simulink model "HW6_JamesWilkinson2"  (R2025b)
settings: Solver=VariableStepAuto  StartTime=0.0  StopTime=10  RelTol=1e-3
values from neighbouring files (symbols this model uses):
  Air_mdot = AirFlow(j)    [All_Conditions.m]
  HeatRate = 10^8    (= 100000000)    [All_Conditions.m]    (also in VariedFuelRate.m = HeatRate_vec(i))
libraries: fl_lib x22, nesl_utility x22, SimscapeFluids_lib x2
settings Model: Creator=james  LastModifiedBy=james

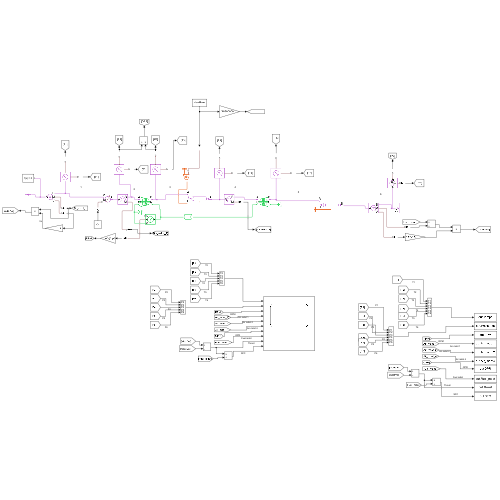
[thumbnail: Simulink's stored preview of the top-level diagram]
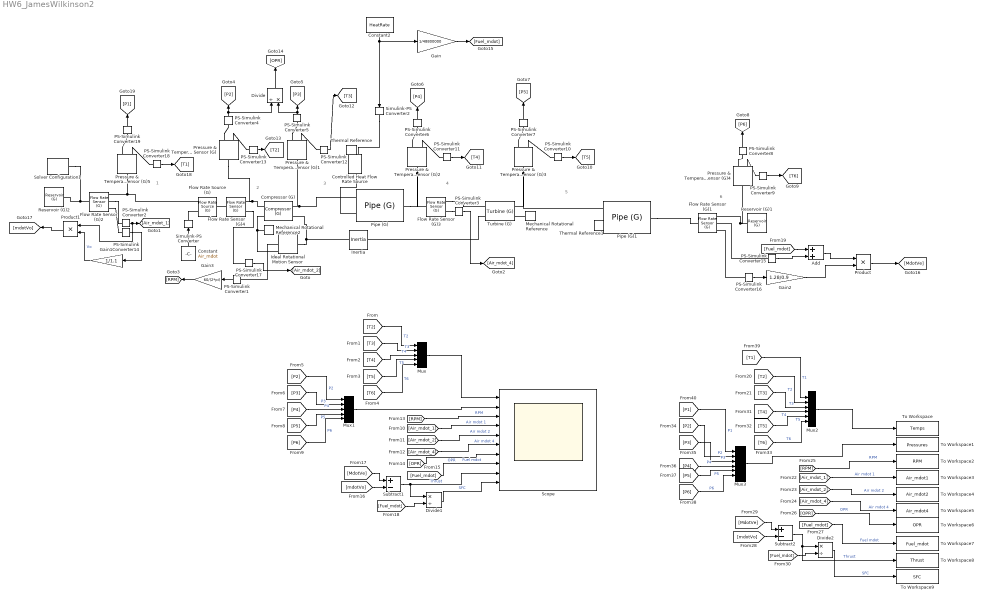
== system HW6_JamesWilkinson2 ==
  note: 6
  note: 5
  note: 4
  note: 3
  note: 2
  note: 1
  Add : Sum
  Compressor (G) : SimscapeFluids_lib/Gas/Turbomachinery/Compressor (G)  parameterization=fluids.gas.turbomachinery.enum.CompressorParameterization.Analytical  NDes=10000 rpm  piDes=DesignedPR  mdotDes=33 kg/s  efficiencyType=fluids.gas.turbomachinery.enum.EfficiencyType.Analytical  efficiencyValue=0.8  etaMax=0.887  etaMin=0.5  mdotMaxEff=30 kg/s  piMaxEff=7  omega_TLU=[5000, 6000, 7000, 7500, 8000, 8500, 9000, 9500, 10000, 11000] rpm  beta_TLU=0 : 1 / 6 : 1  pr_TLU=[1.369, 1.459, 1.587, 1.654, 1.734, 1.775, 1.82; 1.918, 2.075, 2.229, 2.318, 2.405, 2.456, 2.481; 2.706, 2.966, 3.168, 3.334, 3.404, 3.445, 3.435; 3.203, 3.533, 3.833, 4.021, 4.127, 4.135, 4.066; 3.782, 4.222, 4.565, 4.867, 5.065, 5.07, 4.934; 4.302, 4.861, 5.285, 5.821, 6.161, 6.334, 6.142; 4.841, 5.445, 5.988, 6.628, 7.222, 7.623, 7.573; 5.358, 5.997, 6.589, 7.334, 8.012, 8.668, 9; 5.851, 6.491, 7.124, 7.982, 8.754, 9.57, 9.814; 6.707, 7.321, 8.034, 9.047, 9.94, 10.834, 10.998]  mdot_TLU=[10.45, 10.203, 9.784, 9.526, 9.144, 8.947, 8.615; 13.315, 13.018, 12.525, 11.984, 11.455, 11.086, 10.914; 17.601, 17.204, 16.502, 15.8, 14.903, 14.179, 13.184; 20.331, 19.983, 19.39, 18.492, 17.435, 16.293, 14.895; 23.466, 23.092, 22.572, 21.807, 20.687, 19.3, 17.682; 26.295, 26.091, 25.766, 25.28, 24.453, 23.26, 21.311; 29.013, 28.747, 28.641, 28.412, 28.06, 27.098, 25.306; 31.424, 31.379, 31.273, 31.103, 30.849, 30.484, 29.718; 33.688, 33.606, 33.561, 33.513, 33.392, 33.258, 33.059; 37.678, 37.621, 37.575, 37.598, 37.501, 37.415, 37.413] kg/s  eta_TLU=[.68, .69, .695, .7, .701, .705, .704; .7, .725, .75, .755, .745, .73, .725; .77, .795, .81, .805, .78, .765, .745; .795, .812, .825, .82, .805, .78, .75; .82, .837, .848, .849, .835, .805, .78; .83, .845, .856, .86, .855, .84, .8; .83, .848, .859, .869, .86, .852, .83; .828, .845, .857, .869, .862, .855, .85; .806, .83, .85, .86, .859, .857, .853; .79, .8, .82, .835, .845, .848, .849]  SMFault=simscape.enum.assert.action.none  a=1.5  b=5  k=0.03  c=3  d=4  cCap=15  dCap=1  p_reference=0.101325 MPa  T_reference=288.15 K  mechanical_efficiency=0.9  area_A=1.28 m^2  area_B=1 m^2
      settings: InternalSimscapePortConfiguration="{\"Bottom\":[],\"Left\":[{\"id\":\"A\",\"label\":\"A\",\"type\":\"foundation.gas.gas\"},{\"id\":\"C\",\"label\":\"C\",\"type\":\"foundation.mechanical.rotational.rotational\"}],\"Right\":[{\"id\":\"B\",\"label\":\"B\",\"type\":\"foundation.gas.gas\"},{\"id\":\"R\",\"label\":\"R\",\"type\":\"foundation.mechanical.rotational.rotational\"}],\"Top\":[]}"
  Constant : Constant  Value=Air_mdot
  Constant2 : Constant  Value=HeatRate
  Controlled Heat Flow Rate Source : fl_lib/Thermal/Thermal Sources/Controlled Heat Flow Rate Source
  Divide : Product  Inputs=/*
  Divide1 : Product  Inputs=*/
  Divide2 : Product  Inputs=*/
  Flow Rate Sensor (G)1 : fl_lib/Gas/Sensors/Flow Rate Sensor (G)  mass_flow_measure=true  volumetric_flow_measure=true  volumetric_flow_conditions=foundation.enum.volumetric_flow_conditions.actual  p_std=0.101325 MPa  T_std=20 degC  energy_flow_measure=false
      settings: InternalSimscapePortConfiguration="{\"Bottom\":[],\"Left\":[{\"id\":\"A\",\"label\":\"A\",\"type\":\"foundation.gas.gas\"}],\"Right\":[{\"id\":\"B\",\"label\":\"B\",\"type\":\"foundation.gas.gas\"},{\"id\":\"M\",\"label\":\"M\",\"type\":\"output\"},{\"id\":\"V\",\"label\":\"V\",\"type\":\"output\"}],\"Top\":[]}"
  Flow Rate Sensor (G)2 : fl_lib/Gas/Sensors/Flow Rate Sensor (G)  mass_flow_measure=true  volumetric_flow_measure=true  volumetric_flow_conditions=foundation.enum.volumetric_flow_conditions.actual  p_std=0.101325 MPa  T_std=20 degC  energy_flow_measure=false
      settings: InternalSimscapePortConfiguration="{\"Bottom\":[],\"Left\":[{\"id\":\"A\",\"label\":\"A\",\"type\":\"foundation.gas.gas\"}],\"Right\":[{\"id\":\"B\",\"label\":\"B\",\"type\":\"foundation.gas.gas\"},{\"id\":\"M\",\"label\":\"M\",\"type\":\"output\"},{\"id\":\"V\",\"label\":\"V\",\"type\":\"output\"}],\"Top\":[]}"
  Flow Rate Sensor (G)3 : fl_lib/Gas/Sensors/Flow Rate Sensor (G)  mass_flow_measure=true  volumetric_flow_measure=false  volumetric_flow_conditions=foundation.enum.volumetric_flow_conditions.actual  p_std=0.101325 MPa  T_std=20 degC  energy_flow_measure=false
      settings: InternalSimscapePortConfiguration="{\"Bottom\":[],\"Left\":[{\"id\":\"A\",\"label\":\"A\",\"type\":\"foundation.gas.gas\"}],\"Right\":[{\"id\":\"B\",\"label\":\"B\",\"type\":\"foundation.gas.gas\"},{\"id\":\"M\",\"label\":\"M\",\"type\":\"output\"}],\"Top\":[]}"
  Flow Rate Sensor (G)4 : fl_lib/Gas/Sensors/Flow Rate Sensor (G)  mass_flow_measure=true  volumetric_flow_measure=false  volumetric_flow_conditions=foundation.enum.volumetric_flow_conditions.actual  p_std=0.101325 MPa  T_std=20 degC  energy_flow_measure=false
      settings: InternalSimscapePortConfiguration="{\"Bottom\":[],\"Left\":[{\"id\":\"A\",\"label\":\"A\",\"type\":\"foundation.gas.gas\"}],\"Right\":[{\"id\":\"B\",\"label\":\"B\",\"type\":\"foundation.gas.gas\"},{\"id\":\"M\",\"label\":\"M\",\"type\":\"output\"}],\"Top\":[]}"
  Flow Rate Source (G) : fl_lib/Gas/Sources/Flow Rate Source (G)  source_type=foundation.enum.constant_controlled.controlled  flow_type=foundation.enum.mass_volumetric_flow.mass  mass_flow=0 kg/s  volumetric_flow=0 m^3/s  volumetric_flow_conditions=foundation.enum.volumetric_flow_conditions.actual  p_std=0.101325 MPa  T_std=20 degC  power_spec=foundation.enum.power_spec.isentropic  area_A=1.1 m^2  area_B=1.28 m^2
      settings: InternalSimscapePortConfiguration="{\"Bottom\":[],\"Left\":[{\"id\":\"A\",\"label\":\"A\",\"type\":\"foundation.gas.gas\"},{\"id\":\"M\",\"label\":\"M\",\"type\":\"input\"}],\"Right\":[{\"id\":\"B\",\"label\":\"B\",\"type\":\"foundation.gas.gas\"}],\"Top\":[]}"
  Gain : Gain  Gain=1/48800000
  Gain1 : Gain  Gain=1/1.1
  Gain2 : Gain  Gain=1.28/0.9
  Gain3 : Gain  Gain=60/(2*pi)
  Ideal Rotational Motion Sensor : fl_lib/Mechanical/Mechanical Sensors/Ideal Rotational Motion Sensor  reference=foundation.enum.MeasurementReference.difference  acceleration_port=false  velocity_port=true  position_port=true  wrap_angle=false  offset=0 rad
  Inertia : fl_lib/Mechanical/Rotational Elements/Inertia  inertia=0.01 kg*m^2  num_ports=foundation.enum.numPorts2.two  w_specify=on  w_priority=High  w=1400 rad/s  w_nominal_specify=off  w_nominal_value=1  w_nominal_unit=rad/s  t_specify=off  t_priority=None  t=0 N*m  t_nominal_specify=off  t_nominal_value=1  t_nominal_unit=N*m
      settings: InternalSimscapePortConfiguration="{\"Bottom\":[],\"Left\":[{\"id\":\"I\",\"label\":\"\",\"type\":\"foundation.mechanical.rotational.rotational\"}],\"Right\":[{\"id\":\"J\",\"label\":\"\",\"type\":\"foundation.mechanical.rotational.rotational\"}],\"Top\":[]}"
  Mechanical Rotational Reference : fl_lib/Mechanical/Rotational Elements/Mechanical Rotational Reference
  Mechanical Rotational Reference2 : fl_lib/Mechanical/Rotational Elements/Mechanical Rotational Reference
  Mux : Mux  Inputs=5
      settings: DisplayOption=signals
  Mux1 : Mux  Inputs=5
      settings: DisplayOption=signals
  Mux2 : Mux  Inputs=6
      settings: DisplayOption=signals
  Mux3 : Mux  Inputs=6
      settings: DisplayOption=signals
  PS-Simulink Converter{1..19} (19 alike) : nesl_utility/PS-Simulink Converter  PhysicalDomain=network_engine_domain  SubClassName=ps_output  LeftPortType=input  RightPortType=output  PseudoPeriodic=off  Frequencies=[]  VectorFormat=inherit  Unit=inherit  AffineConversion=off
  Pipe (G) : fl_lib/Gas/Elements/Pipe (G)  length=0.5 m  area=1 m^2  Dh=4/(pi) m  length_add=0.1 m  roughness=15e-6 m  Re_lam=2000  Re_tur=4000  shape_factor=64  Nu_lam=3.66  dynamic_compressibility=true  inertia=false  p_init=.5 MPa  p_init_priority=foundation.enum.Priority.High  T_init=500 K  T_init_priority=foundation.enum.Priority.High  mdot_init=0 kg/s  mdot_init_priority=foundation.enum.Priority.High  p_nominal=0.101325 MPa  T_nominal=293.15 K
  Pipe (G)1 : fl_lib/Gas/Elements/Pipe (G)  length=0.5 m  area=1.28 m^2  Dh=sqrt(1.28/pi*4) m  length_add=0.1 m  roughness=15e-6 m  Re_lam=2000  Re_tur=4000  shape_factor=64  Nu_lam=3.66  dynamic_compressibility=true  inertia=false  p_init=0.101325 MPa  p_init_priority=foundation.enum.Priority.High  T_init=293.15 K  T_init_priority=foundation.enum.Priority.High  mdot_init=0 kg/s  mdot_init_priority=foundation.enum.Priority.High  p_nominal=0.101325 MPa  T_nominal=293.15 K
  Pressure & Temperature Sensor (G){,1..5} (6 alike) : fl_lib/Gas/Sensors/Pressure & Temperature Sensor (G)  reference=foundation.enum.MeasurementReference.absolute  pressure=true  pressure_spec=foundation.enum.PressureMeasementSpec.Absolute  temperature=true
      settings: InternalSimscapePortConfiguration="{\"Bottom\":[{\"id\":\"T\",\"label\":\"T\",\"type\":\"output\"}],\"Left\":[{\"id\":\"A\",\"label\":\"A\",\"type\":\"foundation.gas.gas\"}],\"Right\":[{\"id\":\"Pa\",\"label\":\"Pa\",\"type\":\"output\"}],\"Top\":[]}"
  Product : Product
  Product1 : Product
  Reservoir (G)1 : fl_lib/Gas/Elements/Reservoir (G)  pressure_spec=foundation.enum.pressure_spec.specified  reservoir_pressure=Pressure MPa  reservoir_temperature=Temp K  area_A=1.28 m^2
  Reservoir (G)2 : fl_lib/Gas/Elements/Reservoir (G)  pressure_spec=foundation.enum.pressure_spec.specified  reservoir_pressure=Pressure MPa  reservoir_temperature=Temp K  area_A=1.1 m^2
  Scope : Scope  NumInputPorts=10
      settings: ActiveDisplayYMinimum=-67303.986075745488  ActiveDisplayYMaximum=721507.2488354966
  Simulink-PS Converter : nesl_utility/Simulink-PS Converter  PhysicalDomain=network_engine_domain  SubClassName=ps_input  LeftPortType=input  RightPortType=output  PseudoPeriodic=off  Frequencies=[]  NoiseDistribution=none  NoiseParameters=[]  Unit=1  AffineConversion=off  FilteringAndDerivatives=provide  SimscapeFilterOrder=1  InputFilterTimeConstant=0.001  UdotUserProvided=0
  Simulink-PS Converter2 : nesl_utility/Simulink-PS Converter  PhysicalDomain=network_engine_domain  SubClassName=ps_input  LeftPortType=input  RightPortType=output  PseudoPeriodic=off  Frequencies=[]  NoiseDistribution=none  NoiseParameters=[]  Unit=1  AffineConversion=off  FilteringAndDerivatives=provide  SimscapeFilterOrder=1  InputFilterTimeConstant=0.001  UdotUserProvided=0
  Solver Configuration1 : nesl_utility/Solver Configuration  PhysicalDomain=network_engine_domain  SubClassName=solver  LeftPortType=input  RightPortType=generic  Tones=[]  Harmonics=[]  SimulateNoise=off  Profile=off  UseLocalSampling=off  EnableSwitchedLinearOptims=on  FrequencyDomain=off  UseCCode=off  RelTol=0.001  AbsTol=0.001  MinStep=1e-09  ToWorkspace=off  RevertToSquareIcSolve=off  NumHomotopyIterations=100  PhasorMode=off  PhasorModeNumHarmonics=1  ConsistencySolver=NEWTON_XTOL_AFTER_FTOL  IndexReductionMethod=DerivativeReplacement  DoDC=off  ResidualTolerance=1e-09  ConsistencyTolSource=GLOBAL  ConsistencyAbsTol=0.001  ConsistencyRelTol=0.001  ConsistencyTolFactor=0.001  UseLocalSolver=off  LocalSolverChoice=NE_BACKWARD_EULER_ADVANCER  ResolveIndetEquations=on  FunctionEvalNumThread=1  LocalSolverSampleTime=0.001  DoFixedCost=off  MaxNonlinIter=3  MaxModeIter=2  ComputeImpulses=off  ImpulseIterations=2  LinearAlgebra=auto  LinearAlgebraNumThread=0  EquationFormulation=NE_TIME_EF  DelaysMemoryBudget=1024  AutomaticFiltering=on  FilteringTimeConstant=0.001  PartitionStorageMethod=AS_NEEDED  PartitionMemoryBudget=1024  PartitionMethod=ROBUST  MultibodyUseLocalSolver=off  MultibodyLocalSolverChoice=ODE1  MultibodyLocalSolverSampleTime=0.001
  Subtract1 : Sum  Inputs=+-
  Subtract2 : Sum  Inputs=+-
  Thermal Reference : fl_lib/Thermal/Thermal Elements/Thermal Reference
  Thermal Reference1 : fl_lib/Thermal/Thermal Elements/Thermal Reference
  To Workspace : ToWorkspace  VariableName=Temps  SaveFormat=Timeseries  SampleTime=-1
  To Workspace1 : ToWorkspace  VariableName=Pressures  SaveFormat=Timeseries  SampleTime=-1
  To Workspace2 : ToWorkspace  VariableName=RPM  SaveFormat=Timeseries  SampleTime=-1
  To Workspace3 : ToWorkspace  VariableName=Air_mdot1  SaveFormat=Timeseries  SampleTime=-1
  To Workspace4 : ToWorkspace  VariableName=Air_mdot2  SaveFormat=Timeseries  SampleTime=-1
  To Workspace5 : ToWorkspace  VariableName=Air_mdot4  SaveFormat=Timeseries  SampleTime=-1
  To Workspace6 : ToWorkspace  VariableName=OPR  SaveFormat=Timeseries  SampleTime=-1
  To Workspace7 : ToWorkspace  VariableName=Fuel_mdot  SaveFormat=Timeseries  SampleTime=-1
  To Workspace8 : ToWorkspace  VariableName=Thrust  SaveFormat=Timeseries  SampleTime=-1
  To Workspace9 : ToWorkspace  VariableName=SFC  SaveFormat=Timeseries  SampleTime=-1
  Turbine (G) : SimscapeFluids_lib/Gas/Turbomachinery/Turbine (G)  parameterization=fluids.gas.turbomachinery.enum.TurbineParameterization.Analytical  omega_TLU_2=[5000, 6000, 7000, 8000, 9000, 10000, 11000] rpm  variable_nozzle=false  min_nozzle_opening=1e-3  max_nozzle_opening=1  pr_nom=2  mdot_nom=48 kg/s  pr_mdot_TLU=[1.251, 1.345, 1.442, 1.521, 1.596, 1.692, 1.849, 1.972, 2.1, 2.173, 2.259, 2.3424]  mdot_TLU=[39.439, 43.01, 45.556, 46.801, 47.792, 48.388, 48.634, 48.67, 48.689, 48.747, 48.825, 48.912] kg/s  pr_mdot_TLU_2=[1.217, 1.285, 1.323, 1.363, 1.402, 1.427, 1.495, 1.545, 1.6, 1.687, 1.747, 1.8074; 1.231, 1.302, 1.356, 1.404, 1.443, 1.473, 1.525, 1.577, 1.635, 1.709, 1.782, 1.845; 1.242, 1.328, 1.388, 1.437, 1.528, 1.617, 1.704, 1.811, 1.915, 1.979, 2.053, 2.1226; 1.244, 1.339, 1.417, 1.465, 1.528, 1.584, 1.692, 1.787, 1.899, 2, 2.075, 2.1492; 1.245, 1.34, 1.425, 1.492, 1.546, 1.684, 1.748, 1.882, 1.987, 2.084, 2.167, 2.2458; 1.251, 1.345, 1.442, 1.521, 1.596, 1.692, 1.849, 1.972, 2.1, 2.173, 2.259, 2.3424; 1.248, 1.348, 1.447, 1.516, 1.581, 1.651, 1.749, 1.839, 1.93, 2.024, 2.154, 2.242]  mdot_TLU_2=[40.403, 44.417, 46.653, 47.966, 48.97, 49.544, 50.001, 50.081, 50.086, 50.095, 50.09, 50.0922; 40.044, 43.754, 46.125, 47.626, 48.513, 49.105, 49.481, 49.58, 49.597, 49.624, 49.638, 49.633; 39.941, 43.795, 46.017, 47.335, 48.795, 49.199, 49.279, 49.27, 49.248, 49.23, 49.255, 49.2428; 39.896, 43.512, 45.914, 47.061, 48.011, 48.558, 48.943, 49.042, 49.069, 49.01, 49.046, 49.0266; 39.524, 42.934, 45.686, 46.743, 47.715, 48.67, 48.777, 48.836, 48.876, 48.836, 48.845, 48.8184; 39.439, 43.01, 45.556, 46.801, 47.792, 48.388, 48.634, 48.67, 48.639, 48.647, 48.625, 48.5912; 39.502, 42.849, 45.336, 46.385, 47.312, 47.877, 48.222, 48.397, 48.459, 48.482, 48.455, 48.414] kg/s  efficiency_constant=0.8  pr_eta_TLU=[1.252, 1.328, 1.425, 1.544, 1.642, 1.757, 1.873, 2.005, 2.1, 2.204, 2.248, 2.28]  eta_TLU=[.559, .61, .673, .741, .788, .835, .869, .895, .908, .899, .854, .751]  pr_eta_TLU_2=[1.224, 1.246, 1.292, 1.387, 1.457, 1.534, 1.61, 1.686, 1.743, 1.79, 1.871, 1.914; 1.237, 1.25, 1.28, 1.369, 1.459, 1.553, 1.629, 1.716, 1.799, 1.846, 1.927, 1.97; 1.241, 1.255, 1.283, 1.326, 1.401, 1.509, 1.591, 1.704, 1.806, 1.913, 1.994, 2.037; 1.25, 1.265, 1.308, 1.364, 1.456, 1.532, 1.637, 1.739, 1.851, 1.934, 2.042, 2.085; 1.281, 1.314, 1.371, 1.425, 1.498, 1.574, 1.647, 1.749, 1.878, 1.979, 2.091, 2.18; 1.252, 1.328, 1.425, 1.544, 1.642, 1.757, 1.873, 2.005, 2.1, 2.204, 2.248, 2.28; 1.382, 1.43, 1.495, 1.586, 1.688, 1.791, 1.887, 1.99, 2.079, 2.158, 2.249, 2.36]  eta_TLU_2=[.72, .754, .759, .739, .714, .679, .643, .603, .554, .524, .494, .48; .716, .757, .794, .819, .812, .788, .761, .728, .692, .662, .632, .618; .629, .691, .775, .831, .858, .869, .859, .842, .816, .782, .752, .738; .594, .668, .757, .804, .857, .883, .892, .893, .884, .865, .835, .821; .664, .72, .779, .823, .858, .883, .897, .905, .904, .896, .883, .868; .559, .61, .673, .741, .788, .835, .869, .895, .908, .899, .854, .751; .718, .785, .824, .855, .882, .9, .908, .906, .884, .857, .804, .701]  p_reference=0.101325 MPa  T_reference=288.15 K  mechanical_efficiency=0.9  area_A=1 m^2  area_B=1.28 m^2
      settings: InternalSimscapePortConfiguration="{\"Bottom\":[],\"Left\":[{\"id\":\"A\",\"label\":\"A\",\"type\":\"foundation.gas.gas\"},{\"id\":\"R\",\"label\":\"R\",\"type\":\"foundation.mechanical.rotational.rotational\"}],\"Right\":[{\"id\":\"B\",\"label\":\"B\",\"type\":\"foundation.gas.gas\"},{\"id\":\"C\",\"label\":\"C\",\"type\":\"foundation.mechanical.rotational.rotational\"}],\"Top\":[]}"
  wires:
  Constant/1 -> Simulink-PS Converter/1
  PS-Simulink Converter8/1 -> [P6]
  PS-Simulink Converter9/1 -> [T6]
  Add/1 -> Product/1
  Gain2/1 -> Product/2
  PS-Simulink Converter15/1 -> Add/2
  Product/1 -> [MdotVe]
  [Fuel_mdot] -> Add/1
  PS-Simulink Converter16/1 -> Gain2/1
  PS-Simulink Converter10/1 -> [T5]
  PS-Simulink Converter7/1 -> [P5]
  PS-Simulink Converter6/1 -> [P4]
  PS-Simulink Converter11/1 -> [T4]
  PS-Simulink Converter12/1 -> [T3]
  Divide/1 -> [OPR]
  PS-Simulink Converter4/1 -> Divide/1, [P2]
  PS-Simulink Converter5/1 -> Divide/2, [P3]
  PS-Simulink Converter13/1 -> [T2]
  PS-Simulink Converter14/1 -> Gain1/1
  PS-Simulink Converter2/1 -> Product1/1, [Air_mdot_1]
  Gain1/1 -> Product1/2  "Vo"
  Product1/1 -> [mdotVo]
  PS-Simulink Converter1/1 -> Gain3/1
  Gain3/1 -> [RPM]
  PS-Simulink Converter3/1 -> [Air_mdot_4]
  PS-Simulink Converter17/1 -> [Air_mdot_2]
  Subtract1/1 -> Divide1/1, Scope/9  "Thrust"
  [Fuel_mdot] -> Scope/8  "Fuel mdot"
  [Air_mdot_4] -> Scope/6  "Air mdot 4"
  [T3] -> Mux/2  "T3"
  [OPR] -> Scope/7  "OPR"
  [P5] -> Mux1/4  "P5"
  [P2] -> Mux1/1  "P2"
  [T6] -> Mux/5  "T6"
  [MdotVe] -> Subtract1/1
  [mdotVo] -> Subtract1/2
  [T5] -> Mux/4  "T5"
  [Fuel_mdot] -> Divide1/2
  [P3] -> Mux1/2  "P3"
  Divide1/1 -> Scope/10  "SFC"
  [RPM] -> Scope/3  "RPM"
  Mux1/1 -> Scope/2
  [Air_mdot_1] -> Scope/4  "Air mdot 1"
  [T2] -> Mux/1  "T2"
  Mux/1 -> Scope/1
  [T4] -> Mux/3  "T4"
  [Air_mdot_2] -> Scope/5  "Air mdot 2"
  [P6] -> Mux1/5  "P6"
  [P4] -> Mux1/3  "P4"
  Constant2/1 -> Gain/1, Simulink-PS Converter2/1
  Gain/1 -> [Fuel_mdot]
  [Air_mdot_2] -> To Workspace4/1  "Air mdot 2"
  [OPR] -> To Workspace6/1  "OPR"
  [MdotVe] -> Subtract2/1
  [Fuel_mdot] -> Divide2/2
  [P3] -> Mux3/3  "P3"
  [T4] -> Mux2/4  "T4"
  [T2] -> Mux2/2  "T2"
  [P2] -> Mux3/2  "P2"
  [T5] -> Mux2/5  "T5"
  Mux3/1 -> To Workspace1/1
  [T6] -> Mux2/6  "T6"
  Mux2/1 -> To Workspace/1
  Divide2/1 -> To Workspace9/1  "SFC"
  [mdotVo] -> Subtract2/2
  Subtract2/1 -> To Workspace8/1, Divide2/1  "Thrust"
  [Fuel_mdot] -> To Workspace7/1  "Fuel mdot"
  [P6] -> Mux3/6  "P6"
  [P4] -> Mux3/4  "P4"
  [RPM] -> To Workspace2/1  "RPM"
  [Air_mdot_4] -> To Workspace5/1  "Air mdot 4"
  [P5] -> Mux3/5  "P5"
  [Air_mdot_1] -> To Workspace3/1  "Air mdot 1"
  [T3] -> Mux2/3  "T3"
  PS-Simulink Converter18/1 -> [T1]
  PS-Simulink Converter19/1 -> [P1]
  [P1] -> Mux3/1  "P1"
  [T1] -> Mux2/1  "T1"
  connections:
  Mechanical Rotational Reference/LConn1 -- Turbine (G)/RConn2
  Turbine (G)/LConn2 -- Inertia/LConn1
  Flow Rate Source (G)/LConn1 -- Flow Rate Sensor (G)2/RConn1 -- Pressure & Temperature Sensor (G)5/LConn1
  Mechanical Rotational Reference2/LConn1 -- Compressor (G)/LConn2 -- Ideal Rotational Motion Sensor/RConn1
  Inertia/RConn1 -- Compressor (G)/RConn2 -- Ideal Rotational Motion Sensor/LConn1
  Flow Rate Sensor (G)3/RConn1 -- Turbine (G)/LConn1
  Pipe (G)/LConn1 -- Pressure & Temperature Sensor (G)1/LConn1 -- Compressor (G)/RConn1
  Thermal Reference/LConn1 -- Controlled Heat Flow Rate Source/RConn2
  Pipe (G)/LConn2 -- Controlled Heat Flow Rate Source/LConn1
  Simulink-PS Converter2/RConn1 -- Controlled Heat Flow Rate Source/RConn1
  Ideal Rotational Motion Sensor/RConn2 -- PS-Simulink Converter1/LConn1
  Compressor (G)/LConn1 -- Pressure & Temperature Sensor (G)/LConn1 -- Flow Rate Sensor (G)4/RConn1
  Simulink-PS Converter/RConn1 -- Flow Rate Source (G)/LConn2
  Pressure & Temperature Sensor (G)3/LConn1 -- Pipe (G)1/LConn1 -- Turbine (G)/RConn1
  Pipe (G)1/LConn2 -- Thermal Reference1/LConn1
  Reservoir (G)1/LConn1 -- Pressure & Temperature Sensor (G)4/LConn1 -- Flow Rate Sensor (G)1/RConn1
  Pressure & Temperature Sensor (G)4/RConn1 -- PS-Simulink Converter8/LConn1
  Pressure & Temperature Sensor (G)4/RConn2 -- PS-Simulink Converter9/LConn1
  Pipe (G)1/RConn1 -- Flow Rate Sensor (G)1/LConn1
  PS-Simulink Converter15/LConn1 -- Flow Rate Sensor (G)1/RConn2
  PS-Simulink Converter16/LConn1 -- Flow Rate Sensor (G)1/RConn3
  Pressure & Temperature Sensor (G)3/RConn2 -- PS-Simulink Converter10/LConn1
  Pressure & Temperature Sensor (G)3/RConn1 -- PS-Simulink Converter7/LConn1
  Pressure & Temperature Sensor (G)2/RConn2 -- PS-Simulink Converter11/LConn1
  Pressure & Temperature Sensor (G)2/RConn1 -- PS-Simulink Converter6/LConn1
  Pressure & Temperature Sensor (G)1/RConn2 -- PS-Simulink Converter12/LConn1
  Pressure & Temperature Sensor (G)1/RConn1 -- PS-Simulink Converter5/LConn1
  Pressure & Temperature Sensor (G)/RConn2 -- PS-Simulink Converter13/LConn1
  Pressure & Temperature Sensor (G)/RConn1 -- PS-Simulink Converter4/LConn1
  Flow Rate Sensor (G)2/RConn3 -- PS-Simulink Converter14/LConn1
  Flow Rate Sensor (G)2/RConn2 -- PS-Simulink Converter2/LConn1
  Flow Rate Sensor (G)2/LConn1 -- Reservoir (G)2/LConn1 -- Solver Configuration1/RConn1
  Flow Rate Sensor (G)3/RConn2 -- PS-Simulink Converter3/LConn1
  Pressure & Temperature Sensor (G)2/LConn1 -- Pipe (G)/RConn1 -- Flow Rate Sensor (G)3/LConn1
  Flow Rate Sensor (G)4/RConn2 -- PS-Simulink Converter17/LConn1
  Flow Rate Sensor (G)4/LConn1 -- Flow Rate Source (G)/RConn1
  Pressure & Temperature Sensor (G)5/RConn1 -- PS-Simulink Converter19/LConn1
  Pressure & Temperature Sensor (G)5/RConn2 -- PS-Simulink Converter18/LConn1
